simulink library "Water_Tap"  (R2018b)
settings: Solver=ode45  StartTime=0.0  StopTime=10.0  RelTol=1e-3  EnableMultiTasking=on
libraries: carnot x1
settings Model: Creator=lena.frank  LastModifiedBy=P41573
settings DataIOCC: LimitDataPoints=on  SaveFormat=Array  SignalLoggingSaveFormat=ModelDataLogs
settings OptimizationCC: ExpressionDepthLimit=2147483647  LifeSpan=inf
settings DebuggingCC: UnderspecifiedInitializationDetection=Classic  MergeDetectMultiDrivingBlocksExec=none  SolverPrmCheckMsg=warning  FcnCallInpInsideContextMsg=warning  StateNameClashWarn=warning  SFUnexpectedBacktrackingDiag=warning  SFNoUnconditionalDefaultTransitionDiag=warning  SFExecutionAtInitializationDiag=none
settings HardwareCC: ProdBitPerPointer=32  ProdBitPerSizeT=32  ProdBitPerPtrDiffT=32  ProdLargestAtomicFloat=None  ProdIntDivRoundTo=Undefined  ProdEndianess=Unspecified  ProdWordSize=32  ProdHWDeviceType=32-bit Generic
settings ModelReferenceCC: PropagateSignalLabelsOutOfModel=off
settings SFSimCC: SimUseLocalCustomCode=off
settings RTWCC: RTWUseLocalCustomCode=off
settings CodeAppCC: StateflowObjectComments=on
settings GRTTargetCC: TargetLangStandard=C89/C90 (ANSI)  GeneratePreprocessorConditionals=Disable all  CombineOutputUpdateFcns=off  GRTInterface=on
settings ConfigComp: CovMetricSettings=dw  CovHtmlReporting=on  CovSaveCumulativeToWorkspaceVar=on  CovSaveSingleToWorkspaceVar=on  CovExternalEMLEnable=off

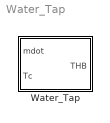
== system Water_Tap ==
  Water_Tap : Subsystem  mask(water tap){dia=0.02, p=2e5}
      mask prompts: dia "diameter at outlet [m]"; p "system pressure [Pa]"
      mask help:
      | The block models a tap, that produces a constant massflow of a fluid at given times.
      | control = 1 is full massflow, control = 0 is no massflow.
      mask init:
      | fluid = 1; %water
      | mix = 0;
      | dia = max(0.001, dia);
      | p = max(p, 0);
      mask Help: eval('man (''water_tap'')')
      mask Display: plot(-10,10,90,90,[44,67,67,45,45,40,40,44],[80,80,72,72,60,60,76,80],[60,45],[90,90],[53,53],[80,90],[24,29,70,75,24],[30,10,10,30,30],[42,42],[32,58],[46,44],[34,54],[38,40],[34,56])

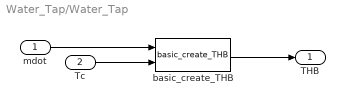
== system Water_Tap/Water_Tap ==
  mdot : Inport
  Tc : Inport  Port=2
  basic_create_THB : carnot/Basic/Hydraulics/basic_create_THB  p=p  fluid=fluid  mix=mix  dia=dia  hgt=0  mID=1
      settings: SourceProductName=Carnot
  THB : Outport
  wires:
  basic_create_THB/1 -> THB/1
  Tc/1 -> basic_create_THB/2
  mdot/1 -> basic_create_THB/1
